simulink model "OL_Adaptive_Integral_Control"  (R2021b)
settings: Solver=ode4  StartTime=0.0  StopTime=60  FixedStep=1e-3  RelTol=1e-3
settings Model: Creator=hellb  LastModifiedBy=hellb
settings SolverCC: AlgebraicLoopSolver=TrustRegion
settings DataIOCC: ReturnWorkspaceOutputs=off
settings DebuggingCC: SFMachineParentedDataDiag=warning  ArithmeticOperatorsInVariantConditions=warning
settings SFSimCC: SimUseLocalCustomCode=off  CustomCodeUndefinedFunction=UseInterfaceOnly
settings RTWCC: RTWUseLocalCustomCode=off

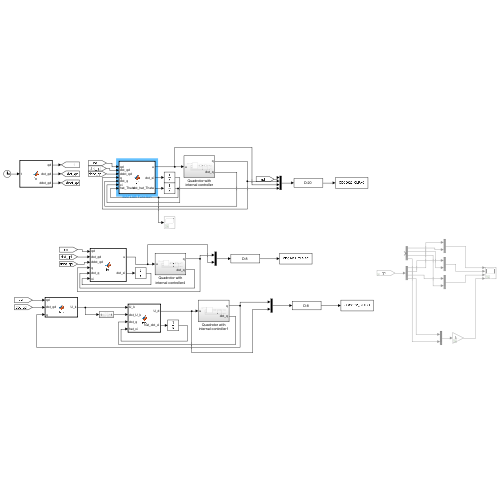
[thumbnail: Simulink's stored preview of the top-level diagram]
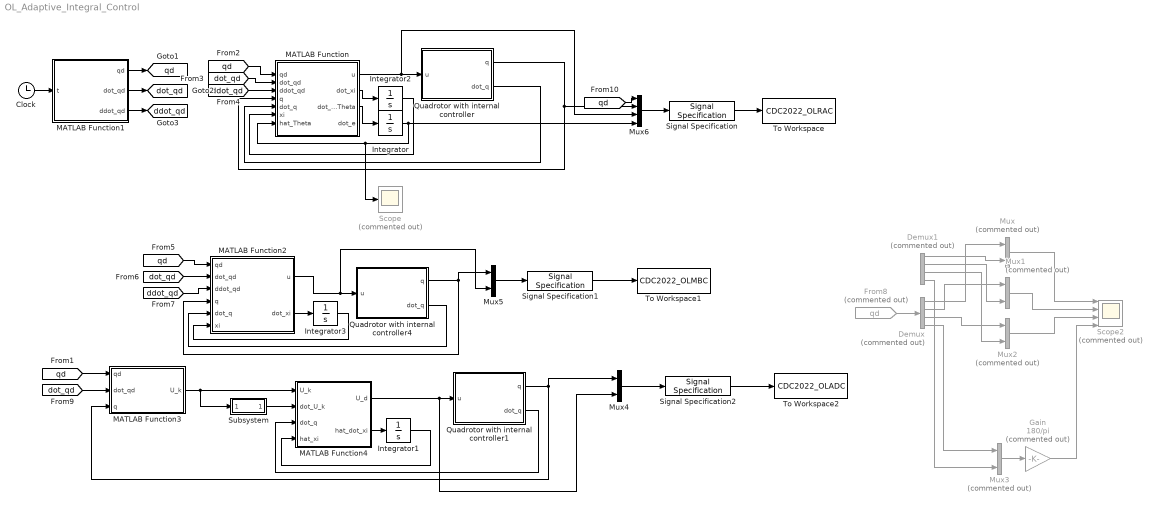
== system OL_Adaptive_Integral_Control ==
  Clock : Clock
  Demux : Demux  Commented=on
  Demux1 : Demux  Commented=on
  From8 : From  Commented=on  GotoTag=qd  TagVisibility=global
  Gain : Gain  Commented=on  Gain=180/pi
  Integrator : Integrator  InitialCondition=0.65*[0.0632; 0.0632; 0.0943; 0.4202; 0.0013; 0.0013; 0.1334; 0.5898]
  Integrator1 : Integrator  InitialCondition=0.65*[0.0632; 0.0632; 0.0943; 0.4202; 0.0013; 0.0013; 0.1334; 0.5898]
  Integrator2 : Integrator  InitialCondition=[0;0;0;0]
  Integrator3 : Integrator  InitialCondition=[0;0;0;0]
  MATLAB Function : MATLAB Function  TreatAsAtomicUnit=on
  MATLAB Function1 : MATLAB Function  TreatAsAtomicUnit=on
  MATLAB Function2 : MATLAB Function  TreatAsAtomicUnit=on
  MATLAB Function3 : MATLAB Function  TreatAsAtomicUnit=on
  MATLAB Function4 : MATLAB Function  TreatAsAtomicUnit=on
  Mux{,1..3} (4 alike) : Mux  Commented=on  Inputs=2
  Mux4 : Mux  Inputs=2
  Mux5 : Mux  Inputs=2
  Mux6 : Mux
  Quadrotor with internal controller : Subsystem
  Quadrotor with internal controller1 : Subsystem
  Quadrotor with internal controller4 : Subsystem
  Scope : Scope  Commented=on
  Scope2 : Scope  Commented=on  NumInputPorts=4
  Signal Specification : SignalSpecification  Dimensions=20
  Signal Specification1 : SignalSpecification  Dimensions=8
  Signal Specification2 : SignalSpecification  Dimensions=8
  Subsystem : Subsystem
  To Workspace : ToWorkspace  VariableName=CDC2022_OLRAC  SaveFormat=Structure With Time  SampleTime=-1
  To Workspace1 : ToWorkspace  VariableName=CDC2022_OLMBC  SaveFormat=Structure With Time  SampleTime=-1
  To Workspace2 : ToWorkspace  VariableName=CDC2022_OLADC  SaveFormat=Structure With Time  SampleTime=-1
  tag scope: ddot_qd=global, dot_qd=global, qd=global
  wires:
  Clock/1 -> MATLAB Function1/1(t)
  MATLAB Function/1(u) -> Mux6/3, Quadrotor with internal controller/1(u)
  Quadrotor with internal controller/1(q) -> MATLAB Function/4(q), Mux6/2
  MATLAB Function/3(dot_hat_Theta) -> Integrator/1
  Integrator/1 -> Mux6/4, Scope/1, MATLAB Function/7(hat_Theta)
  Demux/1 -> Mux/1
  Demux1/1 -> Mux/2
  Mux1/1 -> Scope2/2
  Demux/2 -> Mux1/1
  Demux/3 -> Mux2/1
  Mux3/1 -> Gain/1
  Demux/4 -> Mux3/1
  Quadrotor with internal controller/2(dot_q) -> MATLAB Function/5(dot_q)
  Demux1/3 -> Mux2/2
  Mux2/1 -> Scope2/3
  Demux1/4 -> Mux3/2
  Gain/1 -> Scope2/4
  Mux/1 -> Scope2/1
  Demux1/2 -> Mux1/2
  MATLAB Function2/1(u) -> Mux5/2, Quadrotor with internal controller4/1(u)
  Quadrotor with internal controller4/2(dot_q) -> MATLAB Function2/5(dot_q)
  Quadrotor with internal controller4/1(q) -> Mux5/1, MATLAB Function2/4(q)
  MATLAB Function1/1(qd) -> [qd]
  MATLAB Function1/3(ddot_qd) -> [ddot_qd]
  MATLAB Function1/2(dot_qd) -> [dot_qd]
  [qd] -> MATLAB Function/1(qd)
  [dot_qd] -> MATLAB Function/2(dot_qd)
  [ddot_qd] -> MATLAB Function/3(ddot_qd)
  [ddot_qd] -> MATLAB Function2/3(ddot_qd)
  [dot_qd] -> MATLAB Function2/2(dot_qd)
  [qd] -> MATLAB Function2/1(qd)
  From8/1 -> Demux/1
  MATLAB Function3/1(U_k) -> Subsystem/1(In1), MATLAB Function4/1(U_k)
  Subsystem/1(Out1) -> MATLAB Function4/2(dot_U_k)
  MATLAB Function4/2(hat_dot_xi) -> Integrator1/1
  Integrator1/1 -> MATLAB Function4/4(hat_xi)
  MATLAB Function4/1(U_d) -> Mux4/2, Quadrotor with internal controller1/1(u)
  Quadrotor with internal controller1/2(dot_q) -> MATLAB Function4/3(dot_q)
  Quadrotor with internal controller1/1(q) -> Mux4/1, MATLAB Function3/3(q)
  [qd] -> MATLAB Function3/1(qd)
  [dot_qd] -> MATLAB Function3/2(dot_qd)
  MATLAB Function/2(dot_xi) -> Integrator2/1
  Integrator2/1 -> MATLAB Function/6(xi)
  MATLAB Function2/2(dot_xi) -> Integrator3/1
  Integrator3/1 -> MATLAB Function2/6(xi)
  Mux4/1 -> Signal Specification2/1
  Mux5/1 -> Signal Specification1/1
  Mux6/1 -> Signal Specification/1
  [qd] -> Mux6/1
  Signal Specification/1 -> To Workspace/1
  Signal Specification1/1 -> To Workspace1/1
  Signal Specification2/1 -> To Workspace2/1

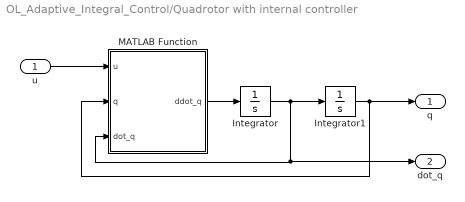
== system OL_Adaptive_Integral_Control/Quadrotor with internal controller ==
  u : Inport
  Integrator : Integrator  InitialCondition=[0;0;0;0]
  Integrator1 : Integrator  InitialCondition=[0;0;0.3;0]
  MATLAB Function : MATLAB Function  TreatAsAtomicUnit=on
  q : Outport  VectorParamsAs1DForOutWhenUnconnected=off
  dot_q : Outport  Port=2  VectorParamsAs1DForOutWhenUnconnected=off
  wires:
  Integrator/1 -> dot_q/1, MATLAB Function/3(dot_q), Integrator1/1
  Integrator1/1 -> q/1, MATLAB Function/2(q)
  MATLAB Function/1(ddot_q) -> Integrator/1
  u/1 -> MATLAB Function/1(u)

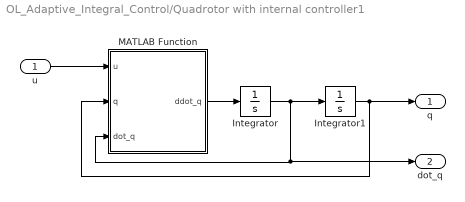
== system OL_Adaptive_Integral_Control/Quadrotor with internal controller1 ==
  u : Inport
  Integrator : Integrator  InitialCondition=[0;0;0;0]
  Integrator1 : Integrator  InitialCondition=[0;0;0.3;0]
  MATLAB Function : MATLAB Function  TreatAsAtomicUnit=on
  q : Outport  VectorParamsAs1DForOutWhenUnconnected=off
  dot_q : Outport  Port=2  VectorParamsAs1DForOutWhenUnconnected=off
  wires:
  Integrator/1 -> dot_q/1, MATLAB Function/3(dot_q), Integrator1/1
  Integrator1/1 -> q/1, MATLAB Function/2(q)
  MATLAB Function/1(ddot_q) -> Integrator/1
  u/1 -> MATLAB Function/1(u)

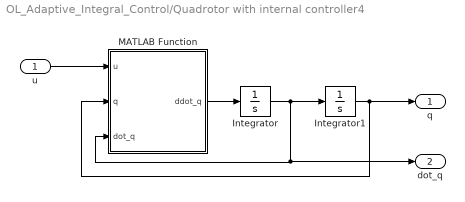
== system OL_Adaptive_Integral_Control/Quadrotor with internal controller4 ==
  u : Inport
  Integrator : Integrator  InitialCondition=[0;0;0;0]
  Integrator1 : Integrator  InitialCondition=[0;0;0.3;0]
  MATLAB Function : MATLAB Function  TreatAsAtomicUnit=on
  q : Outport  VectorParamsAs1DForOutWhenUnconnected=off
  dot_q : Outport  Port=2  VectorParamsAs1DForOutWhenUnconnected=off
  wires:
  Integrator/1 -> dot_q/1, MATLAB Function/3(dot_q), Integrator1/1
  Integrator1/1 -> q/1, MATLAB Function/2(q)
  MATLAB Function/1(ddot_q) -> Integrator/1
  u/1 -> MATLAB Function/1(u)

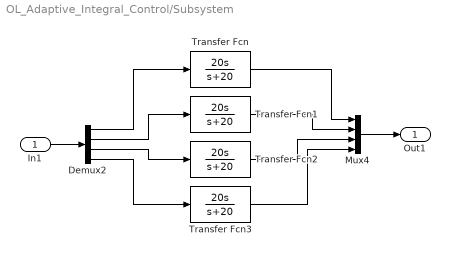
== system OL_Adaptive_Integral_Control/Subsystem ==
  In1 : Inport
  Demux2 : Demux
  Mux4 : Mux
  Transfer Fcn{,1..3} (4 alike) : TransferFcn  Numerator=[20 0]  Denominator=[1 20]
  Out1 : Outport
  wires:
  In1/1 -> Demux2/1
  Mux4/1 -> Out1/1
  Demux2/3 -> Transfer Fcn2/1
  Demux2/2 -> Transfer Fcn1/1
  Demux2/4 -> Transfer Fcn3/1
  Demux2/1 -> Transfer Fcn/1
  Transfer Fcn3/1 -> Mux4/4
  Transfer Fcn2/1 -> Mux4/3
  Transfer Fcn1/1 -> Mux4/2
  Transfer Fcn/1 -> Mux4/1

== matlab function OL_Adaptive_Integral_Control/MATLAB Function ==
  data: qd input; u output; dot_xi output; dot_qd input; ddot_qd input; q input; dot_q input; xi input; dot_hat_Theta output; hat_Theta input; dot_e output
function [u, dot_xi, dot_hat_Theta, dot_e] = fcn(qd, dot_qd, ddot_qd, q, dot_q, xi, hat_Theta)

K_P = diag([1.5 1.5 3.5 2.5]);
Ks = 0.25*K_P;
Ki = 1*diag([0.001 0.001 0.002 0.001]);

Gamma = Ks\(K_P - Ki);

N  = 1*1.8*diag(ones(8,1));
k  = 1*0.09;

psi   = q(4);
e     = qd - q;
dot_e = dot_qd - dot_q;
s     = Gamma*e + dot_e;
f1    = Gamma*dot_e + ddot_qd;
f2    = dot_qd - dot_e;

T  = [cos(psi)  sin(psi) 0 0
      sin(psi) -cos(psi) 0 0
      0         0        1 0
      0         0        0 1];

Phi = [f1(1) 0 0 0 f2(1) 0 0 0
       0 f1(2) 0 0 0 f2(2) 0 0
       0 0 f1(3) 0 0 0 f2(3) 0
       0 0 0 f1(4) 0 0 0 f2(4)];

u      = T\(Ks*s + Ki*xi + Phi*hat_Theta);
dot_xi = s;
dot_hat_Theta = N*(Phi'*s - k*norm(s)*hat_Theta);

== matlab function OL_Adaptive_Integral_Control/Quadrotor with internal controller/MATLAB Function ==
  data: u input; ddot_q output; q input; dot_q input
function ddot_q = fcn(u, q, dot_q)
psi = q(4);
% Parametros tomados del articulo de Adaptive GRNNC
% correspondientes al QBall 2 de Quanser.
g = 9.81;
m = 1.79;
tht_max = deg2rad(92.35);
phi_max = deg2rad(92.35);
dotz_max = 7.7168;
dotpsi_max = deg2rad(99.2730);
tau_dotz   = 0.728;
tau_dotpsi = 0.728;
dx = 0.02;
dy = 0.02;
dz = 0.04;
dpsi = 0.03;
% %%%%%%%%%%%%%%%%%%%%%%%%%%%%%%%%%%%%%%%%%%%%%%%%%
Ku = diag([g*tht_max g*phi_max dotz_max/tau_dotz dotpsi_max/tau_dotpsi]);
Kv = diag([dx dy ((1/tau_dotz)+dz) ((1/tau_dotpsi)+dpsi)]);

T  = [cos(psi)  sin(psi) 0 0
      sin(psi) -cos(psi) 0 0
      0         0        1 0
      0         0        0 1];
  
ddot_q = T*Ku*u - Kv*dot_q;

== matlab function OL_Adaptive_Integral_Control/MATLAB Function1 ==
  data: t input; qd output; dot_qd output; ddot_qd output

function [qd, dot_qd, ddot_qd] = fcn(t)

xfreq = 2*pi/4;
yfreq = 2*pi/8;
zfreq = 2*pi/8;
psifreq = 2*pi/8;
xamp = 0.5;
yamp = 1;
zamp = 0.1;
psiamp = deg2rad(30);
h = 1;
hf = h - zamp + 0.002477;
h0 = 0.3;
b = 0.05;

if t <= 2*pi
qd = [xamp*sin(xfreq*t)*(1-exp(-0.1*t^3))
      yamp*cos(yfreq*t)*(1-exp(-0.1*t^3))
      hf - exp(-b*t^3)*(hf - h0)
      psiamp*sin(psifreq*t)*(1-exp(-0.1*t^3))];

dot_qd = [3*b*t^2*xamp*exp(-b*t^3)*sin(t*xfreq) - xamp*xfreq*cos(t*xfreq)*(exp(-b*t^3) - 1)
          yamp*yfreq*sin(t*yfreq)*(exp(-b*t^3) - 1) + 3*b*t^2*yamp*exp(-b*t^3)*cos(t*yfreq)
          3*b*t^2*exp(-b*t^3)*(hf - h0)
          3*b*t^2*psiamp*exp(-b*t^3)*sin(t*psifreq) - psiamp*psifreq*cos(t*psifreq)*(exp(-b*t^3) - 1)];
ddot_qd = [xamp*xfreq^2*sin(t*xfreq)*(exp(-b*t^3) - 1) - 9*b^2*t^4*xamp*exp(-b*t^3)*sin(t*xfreq) + 6*b*t*xamp*exp(-b*t^3)*sin(t*xfreq) + 6*b*t^2*xamp*xfreq*exp(-b*t^3)*cos(t*xfreq)
           yamp*yfreq^2*cos(t*yfreq)*(exp(-b*t^3) - 1) - 9*b^2*t^4*yamp*exp(-b*t^3)*cos(t*yfreq) + 6*b*t*yamp*exp(-b*t^3)*cos(t*yfreq) - 6*b*t^2*yamp*yfreq*exp(-b*t^3)*sin(t*yfreq)
           6*b*t*exp(-b*t^3)*(hf - h0) - 9*b^2*t^4*exp(-b*t^3)*(hf - h0)
           psiamp*psifreq^2*sin(t*psifreq)*(exp(-b*t^3) - 1) - 9*b^2*t^4*psiamp*exp(-b*t^3)*sin(t*psifreq) + 6*b*t*psiamp*exp(-b*t^3)*sin(t*psifreq) + 6*b*t^2*psiamp*psifreq*exp(-b*t^3)*cos(t*psifreq)];
else
qd = [xamp*sin(xfreq*t)
      yamp*cos(yfreq*t)
      h + zamp*sin(zfreq*t)
      psiamp*sin(psifreq*t)];

dot_qd = [xfreq*xamp*cos(xfreq*t)
          -yfreq*yamp*sin(yfreq*t)
          zamp*zfreq*cos(t*zfreq)
          psifreq*psiamp*cos(psifreq*t)];
ddot_qd = [-xfreq^2*xamp*sin(xfreq*t)
           -yfreq^2*yamp*cos(yfreq*t)
           -zamp*zfreq^2*sin(t*zfreq)
           -psifreq^2*psiamp*sin(psifreq*t)];
end

== matlab function OL_Adaptive_Integral_Control/MATLAB Function2 ==
  data: qd input; u output; dot_qd input; ddot_qd input; q input; dot_q input; xi input; dot_xi output
function [u, dot_xi]  = fcn(qd, dot_qd, ddot_qd, q, dot_q, xi)

Theta = 0.65*[0.0632; 0.0632; 0.0943; 0.4202; 0.0013; 0.0013; 0.1334; 0.5898];

K_P = diag([1.5 1.5 3.5 2.5]);
Ks = 0.25*K_P;
Ki = 1*diag([0.001 0.001 0.002 0.001]);

Gamma = Ks\(K_P - Ki);

psi   = q(4);
e     = qd - q;
dot_e = dot_qd - dot_q;
s     = Gamma*e + dot_e;
f1    = Gamma*dot_e + ddot_qd;
f2    = dot_qd - dot_e;

T  = [cos(psi)  sin(psi) 0 0
      sin(psi) -cos(psi) 0 0
      0         0        1 0
      0         0        0 1];

Phi = [f1(1) 0 0 0 f2(1) 0 0 0
       0 f1(2) 0 0 0 f2(2) 0 0
       0 0 f1(3) 0 0 0 f2(3) 0
       0 0 0 f1(4) 0 0 0 f2(4)];

u      = T\(Ks*s + Ki*xi + Phi*Theta);
dot_xi = s;

== matlab function OL_Adaptive_Integral_Control/Quadrotor with internal controller1/MATLAB Function ==
  data: u input; ddot_q output; q input; dot_q input
function ddot_q = fcn(u, q, dot_q)
psi = q(4);
% Parametros tomados del articulo de Adaptive GRNNC
% correspondientes al QBall 2 de Quanser.
g = 9.81;
m = 1.79;
tht_max = deg2rad(92.35);
phi_max = deg2rad(92.35);
dotz_max = 7.7168;
dotpsi_max = deg2rad(99.2730);
tau_dotz   = 0.728;
tau_dotpsi = 0.728;
dx = 0.02;
dy = 0.02;
dz = 0.04;
dpsi = 0.03;
% %%%%%%%%%%%%%%%%%%%%%%%%%%%%%%%%%%%%%%%%%%%%%%%%%
Ku = diag([g*tht_max g*phi_max dotz_max/tau_dotz dotpsi_max/tau_dotpsi]);
Kv = diag([dx dy ((1/tau_dotz)+dz) ((1/tau_dotpsi)+dpsi)]);

T  = [cos(psi)  sin(psi) 0 0
      sin(psi) -cos(psi) 0 0
      0         0        1 0
      0         0        0 1];
  
ddot_q = T*Ku*u - Kv*dot_q;

== matlab function OL_Adaptive_Integral_Control/MATLAB Function3 ==
  data: qd input; U_k output; dot_qd input; q input
function U_k = fcn(qd, dot_qd, q)

K1 = 20*diag([1 1 1 1]);
K2 = 10*diag([1 1 1 1]);

psi = q(4);
e   = qd - q;

T  = [cos(psi)  sin(psi) 0 0
      sin(psi) -cos(psi) 0 0
      0         0        1 0
      0         0        0 1];

U_k = T\(dot_qd + K1*tanh(K2*e));

== matlab function OL_Adaptive_Integral_Control/MATLAB Function4 ==
  data: U_k input; dot_U_k input; U_d output; dot_q input; hat_xi input; hat_dot_xi output
function [U_d, hat_dot_xi] = fcn(U_k, dot_U_k, dot_q, hat_xi)

K3 = 5*diag([1 1 1 1]);
B_inv = 0.0005*diag(ones(8,1));

% D     = diag([hat_xi(1) hat_xi(2) hat_xi(3) hat_xi(4)]);
% eta   = diag(dot_q)*[hat_xi(5) hat_xi(6) hat_xi(7) hat_xi(8)]';
% sigma = dot_U_k + Kd*(U_k - dot_q);

g11 = dot_U_k(1) + K3(1)*(U_k(1) - dot_q(1));
g15 = dot_q(1);
g22 = dot_U_k(2) + K3(2)*(U_k(2) - dot_q(2));
g26 = dot_q(2);
g33 = dot_U_k(3) + K3(3)*(U_k(3) - dot_q(3));
g37 = dot_q(3);
g44 = dot_U_k(4) + K3(4)*(U_k(4) - dot_q(4));
g48 = dot_q(4);

G = [g11 0 0 0 g15 0 0 0
     0 g22 0 0 0 g26 0 0
     0 0 g33 0 0 0 g37 0
     0 0 0 g44 0 0 0 g48];

% U_d = D*sigma + eta;
U_d = G*hat_xi;
hat_dot_xi = B_inv*G'*(U_k - dot_q);

== matlab function OL_Adaptive_Integral_Control/Quadrotor with internal controller4/MATLAB Function ==
  data: u input; ddot_q output; q input; dot_q input
function ddot_q = fcn(u, q, dot_q)
psi = q(4);
% Parametros tomados del articulo de Adaptive GRNNC
% correspondientes al QBall 2 de Quanser.
g = 9.81;
m = 1.79;
tht_max = deg2rad(92.35);
phi_max = deg2rad(92.35);
dotz_max = 7.7168;
dotpsi_max = deg2rad(99.2730);
tau_dotz   = 0.728;
tau_dotpsi = 0.728;
dx = 0.02;
dy = 0.02;
dz = 0.04;
dpsi = 0.03;
% %%%%%%%%%%%%%%%%%%%%%%%%%%%%%%%%%%%%%%%%%%%%%%%%%
Ku = diag([g*tht_max g*phi_max dotz_max/tau_dotz dotpsi_max/tau_dotpsi]);
Kv = diag([dx dy ((1/tau_dotz)+dz) ((1/tau_dotpsi)+dpsi)]);

T  = [cos(psi)  sin(psi) 0 0
      sin(psi) -cos(psi) 0 0
      0         0        1 0
      0         0        0 1];
  
ddot_q = T*Ku*u - Kv*dot_q;
